simulink model "thermostat"  (R2014b)
settings: Solver=ode1  StartTime=0.0  StopTime=100  FixedStep=0.0001  MaxStep=0.0001  RelTol=1e-3
(part 2 of 2)

== system thermostat/Thermostat44 ==
  Constant : Constant  Value=10
  Constant1 : Constant  Value=37.78
  Discrete-Time Integrator : DiscreteIntegrator  ExternalReset=either  InitialCondition=25  InitialConditionSetting=State (most efficient)  SampleTime=-1
  Discrete-Time Integrator1 : DiscreteIntegrator  ExternalReset=either  InitialCondition=22.78  InitialConditionSetting=State (most efficient)  SampleTime=-1
  MATLAB Function : MATLAB Function  TreatAsAtomicUnit=on
  MATLAB Function1 : MATLAB Function  TreatAsAtomicUnit=on
  Sum : Sum  Inputs=|+-
  Sum1 : Sum  Inputs=|+-
  high : Constant  Value=25
  low : Constant  Value=22.78
  q : Memory
  wires:
  MATLAB Function/1(qNext) -> q/1
  Constant/1 -> Sum/1
  Sum/1 -> Discrete-Time Integrator/1  "x_dot"
  Discrete-Time Integrator1/1 -> MATLAB Function1/2(in1)
  Constant1/1 -> Sum1/1
  Sum1/1 -> Discrete-Time Integrator1/1  "x_dot"
  Discrete-Time Integrator/1 -> MATLAB Function1/1(in0)
  MATLAB Function1/1(out) -> Sum/2, MATLAB Function/1(x), Sum1/2  "x"
  low/1 -> MATLAB Function/3(LOW)
  high/1 -> MATLAB Function/4(HIGH)
  q/1 -> MATLAB Function1/3(ctrl), Discrete-Time Integrator1/2, Discrete-Time Integrator/2, MATLAB Function/2(q)

== system thermostat/Thermostat45 ==
  Constant : Constant  Value=10
  Constant1 : Constant  Value=37.78
  Discrete-Time Integrator : DiscreteIntegrator  ExternalReset=either  InitialCondition=25  InitialConditionSetting=State (most efficient)  SampleTime=-1
  Discrete-Time Integrator1 : DiscreteIntegrator  ExternalReset=either  InitialCondition=22.78  InitialConditionSetting=State (most efficient)  SampleTime=-1
  MATLAB Function : MATLAB Function  TreatAsAtomicUnit=on
  MATLAB Function1 : MATLAB Function  TreatAsAtomicUnit=on
  Sum : Sum  Inputs=|+-
  Sum1 : Sum  Inputs=|+-
  high : Constant  Value=25
  low : Constant  Value=22.78
  q : Memory
  wires:
  MATLAB Function/1(qNext) -> q/1
  Constant/1 -> Sum/1
  Sum/1 -> Discrete-Time Integrator/1  "x_dot"
  Discrete-Time Integrator1/1 -> MATLAB Function1/2(in1)
  Constant1/1 -> Sum1/1
  Sum1/1 -> Discrete-Time Integrator1/1  "x_dot"
  Discrete-Time Integrator/1 -> MATLAB Function1/1(in0)
  MATLAB Function1/1(out) -> Sum/2, MATLAB Function/1(x), Sum1/2  "x"
  low/1 -> MATLAB Function/3(LOW)
  high/1 -> MATLAB Function/4(HIGH)
  q/1 -> MATLAB Function1/3(ctrl), Discrete-Time Integrator1/2, Discrete-Time Integrator/2, MATLAB Function/2(q)

== system thermostat/Thermostat46 ==
  Constant : Constant  Value=10
  Constant1 : Constant  Value=37.78
  Discrete-Time Integrator : DiscreteIntegrator  ExternalReset=either  InitialCondition=25  InitialConditionSetting=State (most efficient)  SampleTime=-1
  Discrete-Time Integrator1 : DiscreteIntegrator  ExternalReset=either  InitialCondition=22.78  InitialConditionSetting=State (most efficient)  SampleTime=-1
  MATLAB Function : MATLAB Function  TreatAsAtomicUnit=on
  MATLAB Function1 : MATLAB Function  TreatAsAtomicUnit=on
  Sum : Sum  Inputs=|+-
  Sum1 : Sum  Inputs=|+-
  high : Constant  Value=25
  low : Constant  Value=22.78
  q : Memory
  wires:
  MATLAB Function/1(qNext) -> q/1
  Constant/1 -> Sum/1
  Sum/1 -> Discrete-Time Integrator/1  "x_dot"
  Discrete-Time Integrator1/1 -> MATLAB Function1/2(in1)
  Constant1/1 -> Sum1/1
  Sum1/1 -> Discrete-Time Integrator1/1  "x_dot"
  Discrete-Time Integrator/1 -> MATLAB Function1/1(in0)
  MATLAB Function1/1(out) -> Sum/2, MATLAB Function/1(x), Sum1/2  "x"
  low/1 -> MATLAB Function/3(LOW)
  high/1 -> MATLAB Function/4(HIGH)
  q/1 -> MATLAB Function1/3(ctrl), Discrete-Time Integrator1/2, Discrete-Time Integrator/2, MATLAB Function/2(q)

== system thermostat/Thermostat47 ==
  Constant : Constant  Value=10
  Constant1 : Constant  Value=37.78
  Discrete-Time Integrator : DiscreteIntegrator  ExternalReset=either  InitialCondition=25  InitialConditionSetting=State (most efficient)  SampleTime=-1
  Discrete-Time Integrator1 : DiscreteIntegrator  ExternalReset=either  InitialCondition=22.78  InitialConditionSetting=State (most efficient)  SampleTime=-1
  MATLAB Function : MATLAB Function  TreatAsAtomicUnit=on
  MATLAB Function1 : MATLAB Function  TreatAsAtomicUnit=on
  Sum : Sum  Inputs=|+-
  Sum1 : Sum  Inputs=|+-
  high : Constant  Value=25
  low : Constant  Value=22.78
  q : Memory
  wires:
  MATLAB Function/1(qNext) -> q/1
  Constant/1 -> Sum/1
  Sum/1 -> Discrete-Time Integrator/1  "x_dot"
  Discrete-Time Integrator1/1 -> MATLAB Function1/2(in1)
  Constant1/1 -> Sum1/1
  Sum1/1 -> Discrete-Time Integrator1/1  "x_dot"
  Discrete-Time Integrator/1 -> MATLAB Function1/1(in0)
  MATLAB Function1/1(out) -> Sum/2, MATLAB Function/1(x), Sum1/2  "x"
  low/1 -> MATLAB Function/3(LOW)
  high/1 -> MATLAB Function/4(HIGH)
  q/1 -> MATLAB Function1/3(ctrl), Discrete-Time Integrator1/2, Discrete-Time Integrator/2, MATLAB Function/2(q)

== system thermostat/Thermostat48 ==
  Constant : Constant  Value=10
  Constant1 : Constant  Value=37.78
  Discrete-Time Integrator : DiscreteIntegrator  ExternalReset=either  InitialCondition=25  InitialConditionSetting=State (most efficient)  SampleTime=-1
  Discrete-Time Integrator1 : DiscreteIntegrator  ExternalReset=either  InitialCondition=22.78  InitialConditionSetting=State (most efficient)  SampleTime=-1
  MATLAB Function : MATLAB Function  TreatAsAtomicUnit=on
  MATLAB Function1 : MATLAB Function  TreatAsAtomicUnit=on
  Sum : Sum  Inputs=|+-
  Sum1 : Sum  Inputs=|+-
  high : Constant  Value=25
  low : Constant  Value=22.78
  q : Memory
  wires:
  MATLAB Function/1(qNext) -> q/1
  Constant/1 -> Sum/1
  Sum/1 -> Discrete-Time Integrator/1  "x_dot"
  Discrete-Time Integrator1/1 -> MATLAB Function1/2(in1)
  Constant1/1 -> Sum1/1
  Sum1/1 -> Discrete-Time Integrator1/1  "x_dot"
  Discrete-Time Integrator/1 -> MATLAB Function1/1(in0)
  MATLAB Function1/1(out) -> Sum/2, MATLAB Function/1(x), Sum1/2  "x"
  low/1 -> MATLAB Function/3(LOW)
  high/1 -> MATLAB Function/4(HIGH)
  q/1 -> MATLAB Function1/3(ctrl), Discrete-Time Integrator1/2, Discrete-Time Integrator/2, MATLAB Function/2(q)

== system thermostat/Thermostat49 ==
  Constant : Constant  Value=10
  Constant1 : Constant  Value=37.78
  Discrete-Time Integrator : DiscreteIntegrator  ExternalReset=either  InitialCondition=25  InitialConditionSetting=State (most efficient)  SampleTime=-1
  Discrete-Time Integrator1 : DiscreteIntegrator  ExternalReset=either  InitialCondition=22.78  InitialConditionSetting=State (most efficient)  SampleTime=-1
  MATLAB Function : MATLAB Function  TreatAsAtomicUnit=on
  MATLAB Function1 : MATLAB Function  TreatAsAtomicUnit=on
  Sum : Sum  Inputs=|+-
  Sum1 : Sum  Inputs=|+-
  high : Constant  Value=25
  low : Constant  Value=22.78
  q : Memory
  wires:
  MATLAB Function/1(qNext) -> q/1
  Constant/1 -> Sum/1
  Sum/1 -> Discrete-Time Integrator/1  "x_dot"
  Discrete-Time Integrator1/1 -> MATLAB Function1/2(in1)
  Constant1/1 -> Sum1/1
  Sum1/1 -> Discrete-Time Integrator1/1  "x_dot"
  Discrete-Time Integrator/1 -> MATLAB Function1/1(in0)
  MATLAB Function1/1(out) -> Sum/2, MATLAB Function/1(x), Sum1/2  "x"
  low/1 -> MATLAB Function/3(LOW)
  high/1 -> MATLAB Function/4(HIGH)
  q/1 -> MATLAB Function1/3(ctrl), Discrete-Time Integrator1/2, Discrete-Time Integrator/2, MATLAB Function/2(q)

== system thermostat/Thermostat5 ==
  Constant : Constant  Value=10
  Constant1 : Constant  Value=37.78
  Discrete-Time Integrator : DiscreteIntegrator  ExternalReset=either  InitialCondition=25  InitialConditionSetting=State (most efficient)  SampleTime=-1
  Discrete-Time Integrator1 : DiscreteIntegrator  ExternalReset=either  InitialCondition=22.78  InitialConditionSetting=State (most efficient)  SampleTime=-1
  MATLAB Function : MATLAB Function  TreatAsAtomicUnit=on
  MATLAB Function1 : MATLAB Function  TreatAsAtomicUnit=on
  Sum : Sum  Inputs=|+-
  Sum1 : Sum  Inputs=|+-
  high : Constant  Value=25
  low : Constant  Value=22.78
  q : Memory
  wires:
  MATLAB Function/1(qNext) -> q/1
  Constant/1 -> Sum/1
  Sum/1 -> Discrete-Time Integrator/1  "x_dot"
  Discrete-Time Integrator1/1 -> MATLAB Function1/2(in1)
  Constant1/1 -> Sum1/1
  Sum1/1 -> Discrete-Time Integrator1/1  "x_dot"
  Discrete-Time Integrator/1 -> MATLAB Function1/1(in0)
  MATLAB Function1/1(out) -> Sum/2, MATLAB Function/1(x), Sum1/2  "x"
  low/1 -> MATLAB Function/3(LOW)
  high/1 -> MATLAB Function/4(HIGH)
  q/1 -> MATLAB Function1/3(ctrl), Discrete-Time Integrator1/2, Discrete-Time Integrator/2, MATLAB Function/2(q)

== system thermostat/Thermostat6 ==
  Constant : Constant  Value=10
  Constant1 : Constant  Value=37.78
  Discrete-Time Integrator : DiscreteIntegrator  ExternalReset=either  InitialCondition=25  InitialConditionSetting=State (most efficient)  SampleTime=-1
  Discrete-Time Integrator1 : DiscreteIntegrator  ExternalReset=either  InitialCondition=22.78  InitialConditionSetting=State (most efficient)  SampleTime=-1
  MATLAB Function : MATLAB Function  TreatAsAtomicUnit=on
  MATLAB Function1 : MATLAB Function  TreatAsAtomicUnit=on
  Sum : Sum  Inputs=|+-
  Sum1 : Sum  Inputs=|+-
  high : Constant  Value=25
  low : Constant  Value=22.78
  q : Memory
  wires:
  MATLAB Function/1(qNext) -> q/1
  Constant/1 -> Sum/1
  Sum/1 -> Discrete-Time Integrator/1  "x_dot"
  Discrete-Time Integrator1/1 -> MATLAB Function1/2(in1)
  Constant1/1 -> Sum1/1
  Sum1/1 -> Discrete-Time Integrator1/1  "x_dot"
  Discrete-Time Integrator/1 -> MATLAB Function1/1(in0)
  MATLAB Function1/1(out) -> Sum/2, MATLAB Function/1(x), Sum1/2  "x"
  low/1 -> MATLAB Function/3(LOW)
  high/1 -> MATLAB Function/4(HIGH)
  q/1 -> MATLAB Function1/3(ctrl), Discrete-Time Integrator1/2, Discrete-Time Integrator/2, MATLAB Function/2(q)

== system thermostat/Thermostat7 ==
  Constant : Constant  Value=10
  Constant1 : Constant  Value=37.78
  Discrete-Time Integrator : DiscreteIntegrator  ExternalReset=either  InitialCondition=25  InitialConditionSetting=State (most efficient)  SampleTime=-1
  Discrete-Time Integrator1 : DiscreteIntegrator  ExternalReset=either  InitialCondition=22.78  InitialConditionSetting=State (most efficient)  SampleTime=-1
  MATLAB Function : MATLAB Function  TreatAsAtomicUnit=on
  MATLAB Function1 : MATLAB Function  TreatAsAtomicUnit=on
  Sum : Sum  Inputs=|+-
  Sum1 : Sum  Inputs=|+-
  high : Constant  Value=25
  low : Constant  Value=22.78
  q : Memory
  wires:
  MATLAB Function/1(qNext) -> q/1
  Constant/1 -> Sum/1
  Sum/1 -> Discrete-Time Integrator/1  "x_dot"
  Discrete-Time Integrator1/1 -> MATLAB Function1/2(in1)
  Constant1/1 -> Sum1/1
  Sum1/1 -> Discrete-Time Integrator1/1  "x_dot"
  Discrete-Time Integrator/1 -> MATLAB Function1/1(in0)
  MATLAB Function1/1(out) -> Sum/2, MATLAB Function/1(x), Sum1/2  "x"
  low/1 -> MATLAB Function/3(LOW)
  high/1 -> MATLAB Function/4(HIGH)
  q/1 -> MATLAB Function1/3(ctrl), Discrete-Time Integrator1/2, Discrete-Time Integrator/2, MATLAB Function/2(q)

== system thermostat/Thermostat8 ==
  Constant : Constant  Value=10
  Constant1 : Constant  Value=37.78
  Discrete-Time Integrator : DiscreteIntegrator  ExternalReset=either  InitialCondition=25  InitialConditionSetting=State (most efficient)  SampleTime=-1
  Discrete-Time Integrator1 : DiscreteIntegrator  ExternalReset=either  InitialCondition=22.78  InitialConditionSetting=State (most efficient)  SampleTime=-1
  MATLAB Function : MATLAB Function  TreatAsAtomicUnit=on
  MATLAB Function1 : MATLAB Function  TreatAsAtomicUnit=on
  Sum : Sum  Inputs=|+-
  Sum1 : Sum  Inputs=|+-
  high : Constant  Value=25
  low : Constant  Value=22.78
  q : Memory
  wires:
  MATLAB Function/1(qNext) -> q/1
  Constant/1 -> Sum/1
  Sum/1 -> Discrete-Time Integrator/1  "x_dot"
  Discrete-Time Integrator1/1 -> MATLAB Function1/2(in1)
  Constant1/1 -> Sum1/1
  Sum1/1 -> Discrete-Time Integrator1/1  "x_dot"
  Discrete-Time Integrator/1 -> MATLAB Function1/1(in0)
  MATLAB Function1/1(out) -> Sum/2, MATLAB Function/1(x), Sum1/2  "x"
  low/1 -> MATLAB Function/3(LOW)
  high/1 -> MATLAB Function/4(HIGH)
  q/1 -> MATLAB Function1/3(ctrl), Discrete-Time Integrator1/2, Discrete-Time Integrator/2, MATLAB Function/2(q)

== system thermostat/Thermostat9 ==
  Constant : Constant  Value=10
  Constant1 : Constant  Value=37.78
  Discrete-Time Integrator : DiscreteIntegrator  ExternalReset=either  InitialCondition=25  InitialConditionSetting=State (most efficient)  SampleTime=-1
  Discrete-Time Integrator1 : DiscreteIntegrator  ExternalReset=either  InitialCondition=22.78  InitialConditionSetting=State (most efficient)  SampleTime=-1
  MATLAB Function : MATLAB Function  TreatAsAtomicUnit=on
  MATLAB Function1 : MATLAB Function  TreatAsAtomicUnit=on
  Sum : Sum  Inputs=|+-
  Sum1 : Sum  Inputs=|+-
  high : Constant  Value=25
  low : Constant  Value=22.78
  q : Memory
  wires:
  MATLAB Function/1(qNext) -> q/1
  Constant/1 -> Sum/1
  Sum/1 -> Discrete-Time Integrator/1  "x_dot"
  Discrete-Time Integrator1/1 -> MATLAB Function1/2(in1)
  Constant1/1 -> Sum1/1
  Sum1/1 -> Discrete-Time Integrator1/1  "x_dot"
  Discrete-Time Integrator/1 -> MATLAB Function1/1(in0)
  MATLAB Function1/1(out) -> Sum/2, MATLAB Function/1(x), Sum1/2  "x"
  low/1 -> MATLAB Function/3(LOW)
  high/1 -> MATLAB Function/4(HIGH)
  q/1 -> MATLAB Function1/3(ctrl), Discrete-Time Integrator1/2, Discrete-Time Integrator/2, MATLAB Function/2(q)

== matlab function thermostat/Thermostat/MATLAB Function1 ==
  data: in0 input; in1 input; ctrl input; out output
function out = select(in0,in1,ctrl)
%#codegen
if(ctrl==0)
    out=in0;
else
    out=in1;
end

== matlab function thermostat/Thermostat/MATLAB Function ==
  data: x input; q input; qNext output; LOW input; HIGH input
function qNext = phi(x,q, LOW, HIGH)
%#codegen
if q==0 && x> LOW
    qNext=0;
elseif q==0 && x <= LOW
    qNext=1;
elseif q==1 && x < HIGH
    qNext=1;
elseif q==1 && x >= HIGH
    qNext=0;
else
    qNext=2; %this should never execute
end

== matlab function thermostat/Thermostat1/MATLAB Function ==
  data: x input; q input; qNext output; LOW input; HIGH input
function qNext = phi(x,q, LOW, HIGH)
%#codegen
if q==0 && x> LOW
    qNext=0;
elseif q==0 && x <= LOW
    qNext=1;
elseif q==1 && x < HIGH
    qNext=1;
elseif q==1 && x >= HIGH
    qNext=0;
else
    qNext=2; %this should never execute
end

== matlab function thermostat/Thermostat1/MATLAB Function1 ==
  data: in0 input; in1 input; ctrl input; out output
function out = select(in0,in1,ctrl)
%#codegen
if(ctrl==0)
    out=in0;
else
    out=in1;
end

== matlab function thermostat/Thermostat2/MATLAB Function ==
  data: x input; q input; qNext output; LOW input; HIGH input
function qNext = phi(x,q, LOW, HIGH)
%#codegen
if q==0 && x> LOW
    qNext=0;
elseif q==0 && x <= LOW
    qNext=1;
elseif q==1 && x < HIGH
    qNext=1;
elseif q==1 && x >= HIGH
    qNext=0;
else
    qNext=2; %this should never execute
end

== matlab function thermostat/Thermostat2/MATLAB Function1 ==
  data: in0 input; in1 input; ctrl input; out output
function out = select(in0,in1,ctrl)
%#codegen
if(ctrl==0)
    out=in0;
else
    out=in1;
end

== matlab function thermostat/Thermostat3/MATLAB Function ==
  data: x input; q input; qNext output; LOW input; HIGH input
function qNext = phi(x,q, LOW, HIGH)
%#codegen
if q==0 && x> LOW
    qNext=0;
elseif q==0 && x <= LOW
    qNext=1;
elseif q==1 && x < HIGH
    qNext=1;
elseif q==1 && x >= HIGH
    qNext=0;
else
    qNext=2; %this should never execute
end

== matlab function thermostat/Thermostat3/MATLAB Function1 ==
  data: in0 input; in1 input; ctrl input; out output
function out = select(in0,in1,ctrl)
%#codegen
if(ctrl==0)
    out=in0;
else
    out=in1;
end

== matlab function thermostat/Thermostat4/MATLAB Function ==
  data: x input; q input; qNext output; LOW input; HIGH input
function qNext = phi(x,q, LOW, HIGH)
%#codegen
if q==0 && x> LOW
    qNext=0;
elseif q==0 && x <= LOW
    qNext=1;
elseif q==1 && x < HIGH
    qNext=1;
elseif q==1 && x >= HIGH
    qNext=0;
else
    qNext=2; %this should never execute
end

== matlab function thermostat/Thermostat4/MATLAB Function1 ==
  data: in0 input; in1 input; ctrl input; out output
function out = select(in0,in1,ctrl)
%#codegen
if(ctrl==0)
    out=in0;
else
    out=in1;
end

== matlab function thermostat/Thermostat5/MATLAB Function ==
  data: x input; q input; qNext output; LOW input; HIGH input
function qNext = phi(x,q, LOW, HIGH)
%#codegen
if q==0 && x> LOW
    qNext=0;
elseif q==0 && x <= LOW
    qNext=1;
elseif q==1 && x < HIGH
    qNext=1;
elseif q==1 && x >= HIGH
    qNext=0;
else
    qNext=2; %this should never execute
end

== matlab function thermostat/Thermostat5/MATLAB Function1 ==
  data: in0 input; in1 input; ctrl input; out output
function out = select(in0,in1,ctrl)
%#codegen
if(ctrl==0)
    out=in0;
else
    out=in1;
end

== matlab function thermostat/Thermostat6/MATLAB Function ==
  data: x input; q input; qNext output; LOW input; HIGH input
function qNext = phi(x,q, LOW, HIGH)
%#codegen
if q==0 && x> LOW
    qNext=0;
elseif q==0 && x <= LOW
    qNext=1;
elseif q==1 && x < HIGH
    qNext=1;
elseif q==1 && x >= HIGH
    qNext=0;
else
    qNext=2; %this should never execute
end

== matlab function thermostat/Thermostat6/MATLAB Function1 ==
  data: in0 input; in1 input; ctrl input; out output
function out = select(in0,in1,ctrl)
%#codegen
if(ctrl==0)
    out=in0;
else
    out=in1;
end

== matlab function thermostat/Thermostat7/MATLAB Function ==
  data: x input; q input; qNext output; LOW input; HIGH input
function qNext = phi(x,q, LOW, HIGH)
%#codegen
if q==0 && x> LOW
    qNext=0;
elseif q==0 && x <= LOW
    qNext=1;
elseif q==1 && x < HIGH
    qNext=1;
elseif q==1 && x >= HIGH
    qNext=0;
else
    qNext=2; %this should never execute
end

== matlab function thermostat/Thermostat7/MATLAB Function1 ==
  data: in0 input; in1 input; ctrl input; out output
function out = select(in0,in1,ctrl)
%#codegen
if(ctrl==0)
    out=in0;
else
    out=in1;
end

== matlab function thermostat/Thermostat8/MATLAB Function ==
  data: x input; q input; qNext output; LOW input; HIGH input
function qNext = phi(x,q, LOW, HIGH)
%#codegen
if q==0 && x> LOW
    qNext=0;
elseif q==0 && x <= LOW
    qNext=1;
elseif q==1 && x < HIGH
    qNext=1;
elseif q==1 && x >= HIGH
    qNext=0;
else
    qNext=2; %this should never execute
end

== matlab function thermostat/Thermostat8/MATLAB Function1 ==
  data: in0 input; in1 input; ctrl input; out output
function out = select(in0,in1,ctrl)
%#codegen
if(ctrl==0)
    out=in0;
else
    out=in1;
end

== matlab function thermostat/Thermostat9/MATLAB Function ==
  data: x input; q input; qNext output; LOW input; HIGH input
function qNext = phi(x,q, LOW, HIGH)
%#codegen
if q==0 && x> LOW
    qNext=0;
elseif q==0 && x <= LOW
    qNext=1;
elseif q==1 && x < HIGH
    qNext=1;
elseif q==1 && x >= HIGH
    qNext=0;
else
    qNext=2; %this should never execute
end

== matlab function thermostat/Thermostat9/MATLAB Function1 ==
  data: in0 input; in1 input; ctrl input; out output
function out = select(in0,in1,ctrl)
%#codegen
if(ctrl==0)
    out=in0;
else
    out=in1;
end

== matlab function thermostat/Thermostat10/MATLAB Function ==
  data: x input; q input; qNext output; LOW input; HIGH input
function qNext = phi(x,q, LOW, HIGH)
%#codegen
if q==0 && x> LOW
    qNext=0;
elseif q==0 && x <= LOW
    qNext=1;
elseif q==1 && x < HIGH
    qNext=1;
elseif q==1 && x >= HIGH
    qNext=0;
else
    qNext=2; %this should never execute
end

== matlab function thermostat/Thermostat10/MATLAB Function1 ==
  data: in0 input; in1 input; ctrl input; out output
function out = select(in0,in1,ctrl)
%#codegen
if(ctrl==0)
    out=in0;
else
    out=in1;
end

== matlab function thermostat/Thermostat11/MATLAB Function ==
  data: x input; q input; qNext output; LOW input; HIGH input
function qNext = phi(x,q, LOW, HIGH)
%#codegen
if q==0 && x> LOW
    qNext=0;
elseif q==0 && x <= LOW
    qNext=1;
elseif q==1 && x < HIGH
    qNext=1;
elseif q==1 && x >= HIGH
    qNext=0;
else
    qNext=2; %this should never execute
end

== matlab function thermostat/Thermostat11/MATLAB Function1 ==
  data: in0 input; in1 input; ctrl input; out output
function out = select(in0,in1,ctrl)
%#codegen
if(ctrl==0)
    out=in0;
else
    out=in1;
end

== matlab function thermostat/Thermostat12/MATLAB Function ==
  data: x input; q input; qNext output; LOW input; HIGH input
function qNext = phi(x,q, LOW, HIGH)
%#codegen
if q==0 && x> LOW
    qNext=0;
elseif q==0 && x <= LOW
    qNext=1;
elseif q==1 && x < HIGH
    qNext=1;
elseif q==1 && x >= HIGH
    qNext=0;
else
    qNext=2; %this should never execute
end

== matlab function thermostat/Thermostat12/MATLAB Function1 ==
  data: in0 input; in1 input; ctrl input; out output
function out = select(in0,in1,ctrl)
%#codegen
if(ctrl==0)
    out=in0;
else
    out=in1;
end

== matlab function thermostat/Thermostat13/MATLAB Function ==
  data: x input; q input; qNext output; LOW input; HIGH input
function qNext = phi(x,q, LOW, HIGH)
%#codegen
if q==0 && x> LOW
    qNext=0;
elseif q==0 && x <= LOW
    qNext=1;
elseif q==1 && x < HIGH
    qNext=1;
elseif q==1 && x >= HIGH
    qNext=0;
else
    qNext=2; %this should never execute
end

== matlab function thermostat/Thermostat13/MATLAB Function1 ==
  data: in0 input; in1 input; ctrl input; out output
function out = select(in0,in1,ctrl)
%#codegen
if(ctrl==0)
    out=in0;
else
    out=in1;
end

== matlab function thermostat/Thermostat14/MATLAB Function ==
  data: x input; q input; qNext output; LOW input; HIGH input
function qNext = phi(x,q, LOW, HIGH)
%#codegen
if q==0 && x> LOW
    qNext=0;
elseif q==0 && x <= LOW
    qNext=1;
elseif q==1 && x < HIGH
    qNext=1;
elseif q==1 && x >= HIGH
    qNext=0;
else
    qNext=2; %this should never execute
end

== matlab function thermostat/Thermostat14/MATLAB Function1 ==
  data: in0 input; in1 input; ctrl input; out output
function out = select(in0,in1,ctrl)
%#codegen
if(ctrl==0)
    out=in0;
else
    out=in1;
end

== matlab function thermostat/Thermostat15/MATLAB Function ==
  data: x input; q input; qNext output; LOW input; HIGH input
function qNext = phi(x,q, LOW, HIGH)
%#codegen
if q==0 && x> LOW
    qNext=0;
elseif q==0 && x <= LOW
    qNext=1;
elseif q==1 && x < HIGH
    qNext=1;
elseif q==1 && x >= HIGH
    qNext=0;
else
    qNext=2; %this should never execute
end

== matlab function thermostat/Thermostat15/MATLAB Function1 ==
  data: in0 input; in1 input; ctrl input; out output
function out = select(in0,in1,ctrl)
%#codegen
if(ctrl==0)
    out=in0;
else
    out=in1;
end

== matlab function thermostat/Thermostat16/MATLAB Function ==
  data: x input; q input; qNext output; LOW input; HIGH input
function qNext = phi(x,q, LOW, HIGH)
%#codegen
if q==0 && x> LOW
    qNext=0;
elseif q==0 && x <= LOW
    qNext=1;
elseif q==1 && x < HIGH
    qNext=1;
elseif q==1 && x >= HIGH
    qNext=0;
else
    qNext=2; %this should never execute
end

== matlab function thermostat/Thermostat16/MATLAB Function1 ==
  data: in0 input; in1 input; ctrl input; out output
function out = select(in0,in1,ctrl)
%#codegen
if(ctrl==0)
    out=in0;
else
    out=in1;
end

== matlab function thermostat/Thermostat17/MATLAB Function ==
  data: x input; q input; qNext output; LOW input; HIGH input
function qNext = phi(x,q, LOW, HIGH)
%#codegen
if q==0 && x> LOW
    qNext=0;
elseif q==0 && x <= LOW
    qNext=1;
elseif q==1 && x < HIGH
    qNext=1;
elseif q==1 && x >= HIGH
    qNext=0;
else
    qNext=2; %this should never execute
end

== matlab function thermostat/Thermostat17/MATLAB Function1 ==
  data: in0 input; in1 input; ctrl input; out output
function out = select(in0,in1,ctrl)
%#codegen
if(ctrl==0)
    out=in0;
else
    out=in1;
end

== matlab function thermostat/Thermostat18/MATLAB Function ==
  data: x input; q input; qNext output; LOW input; HIGH input
function qNext = phi(x,q, LOW, HIGH)
%#codegen
if q==0 && x> LOW
    qNext=0;
elseif q==0 && x <= LOW
    qNext=1;
elseif q==1 && x < HIGH
    qNext=1;
elseif q==1 && x >= HIGH
    qNext=0;
else
    qNext=2; %this should never execute
end

== matlab function thermostat/Thermostat18/MATLAB Function1 ==
  data: in0 input; in1 input; ctrl input; out output
function out = select(in0,in1,ctrl)
%#codegen
if(ctrl==0)
    out=in0;
else
    out=in1;
end

== matlab function thermostat/Thermostat19/MATLAB Function ==
  data: x input; q input; qNext output; LOW input; HIGH input
function qNext = phi(x,q, LOW, HIGH)
%#codegen
if q==0 && x> LOW
    qNext=0;
elseif q==0 && x <= LOW
    qNext=1;
elseif q==1 && x < HIGH
    qNext=1;
elseif q==1 && x >= HIGH
    qNext=0;
else
    qNext=2; %this should never execute
end

== matlab function thermostat/Thermostat19/MATLAB Function1 ==
  data: in0 input; in1 input; ctrl input; out output
function out = select(in0,in1,ctrl)
%#codegen
if(ctrl==0)
    out=in0;
else
    out=in1;
end

== matlab function thermostat/Thermostat20/MATLAB Function ==
  data: x input; q input; qNext output; LOW input; HIGH input
function qNext = phi(x,q, LOW, HIGH)
%#codegen
if q==0 && x> LOW
    qNext=0;
elseif q==0 && x <= LOW
    qNext=1;
elseif q==1 && x < HIGH
    qNext=1;
elseif q==1 && x >= HIGH
    qNext=0;
else
    qNext=2; %this should never execute
end

== matlab function thermostat/Thermostat20/MATLAB Function1 ==
  data: in0 input; in1 input; ctrl input; out output
function out = select(in0,in1,ctrl)
%#codegen
if(ctrl==0)
    out=in0;
else
    out=in1;
end

== matlab function thermostat/Thermostat21/MATLAB Function ==
  data: x input; q input; qNext output; LOW input; HIGH input
function qNext = phi(x,q, LOW, HIGH)
%#codegen
if q==0 && x> LOW
    qNext=0;
elseif q==0 && x <= LOW
    qNext=1;
elseif q==1 && x < HIGH
    qNext=1;
elseif q==1 && x >= HIGH
    qNext=0;
else
    qNext=2; %this should never execute
end

== matlab function thermostat/Thermostat21/MATLAB Function1 ==
  data: in0 input; in1 input; ctrl input; out output
function out = select(in0,in1,ctrl)
%#codegen
if(ctrl==0)
    out=in0;
else
    out=in1;
end

== matlab function thermostat/Thermostat22/MATLAB Function ==
  data: x input; q input; qNext output; LOW input; HIGH input
function qNext = phi(x,q, LOW, HIGH)
%#codegen
if q==0 && x> LOW
    qNext=0;
elseif q==0 && x <= LOW
    qNext=1;
elseif q==1 && x < HIGH
    qNext=1;
elseif q==1 && x >= HIGH
    qNext=0;
else
    qNext=2; %this should never execute
end

== matlab function thermostat/Thermostat22/MATLAB Function1 ==
  data: in0 input; in1 input; ctrl input; out output
function out = select(in0,in1,ctrl)
%#codegen
if(ctrl==0)
    out=in0;
else
    out=in1;
end

== matlab function thermostat/Thermostat23/MATLAB Function ==
  data: x input; q input; qNext output; LOW input; HIGH input
function qNext = phi(x,q, LOW, HIGH)
%#codegen
if q==0 && x> LOW
    qNext=0;
elseif q==0 && x <= LOW
    qNext=1;
elseif q==1 && x < HIGH
    qNext=1;
elseif q==1 && x >= HIGH
    qNext=0;
else
    qNext=2; %this should never execute
end

== matlab function thermostat/Thermostat23/MATLAB Function1 ==
  data: in0 input; in1 input; ctrl input; out output
function out = select(in0,in1,ctrl)
%#codegen
if(ctrl==0)
    out=in0;
else
    out=in1;
end

== matlab function thermostat/Thermostat24/MATLAB Function ==
  data: x input; q input; qNext output; LOW input; HIGH input
function qNext = phi(x,q, LOW, HIGH)
%#codegen
if q==0 && x> LOW
    qNext=0;
elseif q==0 && x <= LOW
    qNext=1;
elseif q==1 && x < HIGH
    qNext=1;
elseif q==1 && x >= HIGH
    qNext=0;
else
    qNext=2; %this should never execute
end

== matlab function thermostat/Thermostat24/MATLAB Function1 ==
  data: in0 input; in1 input; ctrl input; out output
function out = select(in0,in1,ctrl)
%#codegen
if(ctrl==0)
    out=in0;
else
    out=in1;
end

== matlab function thermostat/Thermostat25/MATLAB Function ==
  data: x input; q input; qNext output; LOW input; HIGH input
function qNext = phi(x,q, LOW, HIGH)
%#codegen
if q==0 && x> LOW
    qNext=0;
elseif q==0 && x <= LOW
    qNext=1;
elseif q==1 && x < HIGH
    qNext=1;
elseif q==1 && x >= HIGH
    qNext=0;
else
    qNext=2; %this should never execute
end

== matlab function thermostat/Thermostat25/MATLAB Function1 ==
  data: in0 input; in1 input; ctrl input; out output
function out = select(in0,in1,ctrl)
%#codegen
if(ctrl==0)
    out=in0;
else
    out=in1;
end

== matlab function thermostat/Thermostat26/MATLAB Function ==
  data: x input; q input; qNext output; LOW input; HIGH input
function qNext = phi(x,q, LOW, HIGH)
%#codegen
if q==0 && x> LOW
    qNext=0;
elseif q==0 && x <= LOW
    qNext=1;
elseif q==1 && x < HIGH
    qNext=1;
elseif q==1 && x >= HIGH
    qNext=0;
else
    qNext=2; %this should never execute
end

== matlab function thermostat/Thermostat26/MATLAB Function1 ==
  data: in0 input; in1 input; ctrl input; out output
function out = select(in0,in1,ctrl)
%#codegen
if(ctrl==0)
    out=in0;
else
    out=in1;
end

== matlab function thermostat/Thermostat27/MATLAB Function ==
  data: x input; q input; qNext output; LOW input; HIGH input
function qNext = phi(x,q, LOW, HIGH)
%#codegen
if q==0 && x> LOW
    qNext=0;
elseif q==0 && x <= LOW
    qNext=1;
elseif q==1 && x < HIGH
    qNext=1;
elseif q==1 && x >= HIGH
    qNext=0;
else
    qNext=2; %this should never execute
end

== matlab function thermostat/Thermostat27/MATLAB Function1 ==
  data: in0 input; in1 input; ctrl input; out output
function out = select(in0,in1,ctrl)
%#codegen
if(ctrl==0)
    out=in0;
else
    out=in1;
end

== matlab function thermostat/Thermostat28/MATLAB Function ==
  data: x input; q input; qNext output; LOW input; HIGH input
function qNext = phi(x,q, LOW, HIGH)
%#codegen
if q==0 && x> LOW
    qNext=0;
elseif q==0 && x <= LOW
    qNext=1;
elseif q==1 && x < HIGH
    qNext=1;
elseif q==1 && x >= HIGH
    qNext=0;
else
    qNext=2; %this should never execute
end

== matlab function thermostat/Thermostat28/MATLAB Function1 ==
  data: in0 input; in1 input; ctrl input; out output
function out = select(in0,in1,ctrl)
%#codegen
if(ctrl==0)
    out=in0;
else
    out=in1;
end

== matlab function thermostat/Thermostat29/MATLAB Function ==
  data: x input; q input; qNext output; LOW input; HIGH input
function qNext = phi(x,q, LOW, HIGH)
%#codegen
if q==0 && x> LOW
    qNext=0;
elseif q==0 && x <= LOW
    qNext=1;
elseif q==1 && x < HIGH
    qNext=1;
elseif q==1 && x >= HIGH
    qNext=0;
else
    qNext=2; %this should never execute
end

== matlab function thermostat/Thermostat29/MATLAB Function1 ==
  data: in0 input; in1 input; ctrl input; out output
function out = select(in0,in1,ctrl)
%#codegen
if(ctrl==0)
    out=in0;
else
    out=in1;
end

== matlab function thermostat/Thermostat30/MATLAB Function ==
  data: x input; q input; qNext output; LOW input; HIGH input
function qNext = phi(x,q, LOW, HIGH)
%#codegen
if q==0 && x> LOW
    qNext=0;
elseif q==0 && x <= LOW
    qNext=1;
elseif q==1 && x < HIGH
    qNext=1;
elseif q==1 && x >= HIGH
    qNext=0;
else
    qNext=2; %this should never execute
end

== matlab function thermostat/Thermostat30/MATLAB Function1 ==
  data: in0 input; in1 input; ctrl input; out output
function out = select(in0,in1,ctrl)
%#codegen
if(ctrl==0)
    out=in0;
else
    out=in1;
end

== matlab function thermostat/Thermostat31/MATLAB Function ==
  data: x input; q input; qNext output; LOW input; HIGH input
function qNext = phi(x,q, LOW, HIGH)
%#codegen
if q==0 && x> LOW
    qNext=0;
elseif q==0 && x <= LOW
    qNext=1;
elseif q==1 && x < HIGH
    qNext=1;
elseif q==1 && x >= HIGH
    qNext=0;
else
    qNext=2; %this should never execute
end

== matlab function thermostat/Thermostat31/MATLAB Function1 ==
  data: in0 input; in1 input; ctrl input; out output
function out = select(in0,in1,ctrl)
%#codegen
if(ctrl==0)
    out=in0;
else
    out=in1;
end

== matlab function thermostat/Thermostat32/MATLAB Function ==
  data: x input; q input; qNext output; LOW input; HIGH input
function qNext = phi(x,q, LOW, HIGH)
%#codegen
if q==0 && x> LOW
    qNext=0;
elseif q==0 && x <= LOW
    qNext=1;
elseif q==1 && x < HIGH
    qNext=1;
elseif q==1 && x >= HIGH
    qNext=0;
else
    qNext=2; %this should never execute
end

== matlab function thermostat/Thermostat32/MATLAB Function1 ==
  data: in0 input; in1 input; ctrl input; out output
function out = select(in0,in1,ctrl)
%#codegen
if(ctrl==0)
    out=in0;
else
    out=in1;
end

== matlab function thermostat/Thermostat33/MATLAB Function ==
  data: x input; q input; qNext output; LOW input; HIGH input
function qNext = phi(x,q, LOW, HIGH)
%#codegen
if q==0 && x> LOW
    qNext=0;
elseif q==0 && x <= LOW
    qNext=1;
elseif q==1 && x < HIGH
    qNext=1;
elseif q==1 && x >= HIGH
    qNext=0;
else
    qNext=2; %this should never execute
end

== matlab function thermostat/Thermostat33/MATLAB Function1 ==
  data: in0 input; in1 input; ctrl input; out output
function out = select(in0,in1,ctrl)
%#codegen
if(ctrl==0)
    out=in0;
else
    out=in1;
end

== matlab function thermostat/Thermostat34/MATLAB Function ==
  data: x input; q input; qNext output; LOW input; HIGH input
function qNext = phi(x,q, LOW, HIGH)
%#codegen
if q==0 && x> LOW
    qNext=0;
elseif q==0 && x <= LOW
    qNext=1;
elseif q==1 && x < HIGH
    qNext=1;
elseif q==1 && x >= HIGH
    qNext=0;
else
    qNext=2; %this should never execute
end

== matlab function thermostat/Thermostat34/MATLAB Function1 ==
  data: in0 input; in1 input; ctrl input; out output
function out = select(in0,in1,ctrl)
%#codegen
if(ctrl==0)
    out=in0;
else
    out=in1;
end

== matlab function thermostat/Thermostat35/MATLAB Function ==
  data: x input; q input; qNext output; LOW input; HIGH input
function qNext = phi(x,q, LOW, HIGH)
%#codegen
if q==0 && x> LOW
    qNext=0;
elseif q==0 && x <= LOW
    qNext=1;
elseif q==1 && x < HIGH
    qNext=1;
elseif q==1 && x >= HIGH
    qNext=0;
else
    qNext=2; %this should never execute
end

== matlab function thermostat/Thermostat35/MATLAB Function1 ==
  data: in0 input; in1 input; ctrl input; out output
function out = select(in0,in1,ctrl)
%#codegen
if(ctrl==0)
    out=in0;
else
    out=in1;
end

== matlab function thermostat/Thermostat36/MATLAB Function ==
  data: x input; q input; qNext output; LOW input; HIGH input
function qNext = phi(x,q, LOW, HIGH)
%#codegen
if q==0 && x> LOW
    qNext=0;
elseif q==0 && x <= LOW
    qNext=1;
elseif q==1 && x < HIGH
    qNext=1;
elseif q==1 && x >= HIGH
    qNext=0;
else
    qNext=2; %this should never execute
end

== matlab function thermostat/Thermostat36/MATLAB Function1 ==
  data: in0 input; in1 input; ctrl input; out output
function out = select(in0,in1,ctrl)
%#codegen
if(ctrl==0)
    out=in0;
else
    out=in1;
end

== matlab function thermostat/Thermostat37/MATLAB Function ==
  data: x input; q input; qNext output; LOW input; HIGH input
function qNext = phi(x,q, LOW, HIGH)
%#codegen
if q==0 && x> LOW
    qNext=0;
elseif q==0 && x <= LOW
    qNext=1;
elseif q==1 && x < HIGH
    qNext=1;
elseif q==1 && x >= HIGH
    qNext=0;
else
    qNext=2; %this should never execute
end

== matlab function thermostat/Thermostat37/MATLAB Function1 ==
  data: in0 input; in1 input; ctrl input; out output
function out = select(in0,in1,ctrl)
%#codegen
if(ctrl==0)
    out=in0;
else
    out=in1;
end

== matlab function thermostat/Thermostat38/MATLAB Function ==
  data: x input; q input; qNext output; LOW input; HIGH input
function qNext = phi(x,q, LOW, HIGH)
%#codegen
if q==0 && x> LOW
    qNext=0;
elseif q==0 && x <= LOW
    qNext=1;
elseif q==1 && x < HIGH
    qNext=1;
elseif q==1 && x >= HIGH
    qNext=0;
else
    qNext=2; %this should never execute
end

== matlab function thermostat/Thermostat38/MATLAB Function1 ==
  data: in0 input; in1 input; ctrl input; out output
function out = select(in0,in1,ctrl)
%#codegen
if(ctrl==0)
    out=in0;
else
    out=in1;
end

== matlab function thermostat/Thermostat39/MATLAB Function ==
  data: x input; q input; qNext output; LOW input; HIGH input
function qNext = phi(x,q, LOW, HIGH)
%#codegen
if q==0 && x> LOW
    qNext=0;
elseif q==0 && x <= LOW
    qNext=1;
elseif q==1 && x < HIGH
    qNext=1;
elseif q==1 && x >= HIGH
    qNext=0;
else
    qNext=2; %this should never execute
end

== matlab function thermostat/Thermostat39/MATLAB Function1 ==
  data: in0 input; in1 input; ctrl input; out output
function out = select(in0,in1,ctrl)
%#codegen
if(ctrl==0)
    out=in0;
else
    out=in1;
end

== matlab function thermostat/Thermostat40/MATLAB Function ==
  data: x input; q input; qNext output; LOW input; HIGH input
function qNext = phi(x,q, LOW, HIGH)
%#codegen
if q==0 && x> LOW
    qNext=0;
elseif q==0 && x <= LOW
    qNext=1;
elseif q==1 && x < HIGH
    qNext=1;
elseif q==1 && x >= HIGH
    qNext=0;
else
    qNext=2; %this should never execute
end

== matlab function thermostat/Thermostat40/MATLAB Function1 ==
  data: in0 input; in1 input; ctrl input; out output
function out = select(in0,in1,ctrl)
%#codegen
if(ctrl==0)
    out=in0;
else
    out=in1;
end

== matlab function thermostat/Thermostat41/MATLAB Function ==
  data: x input; q input; qNext output; LOW input; HIGH input
function qNext = phi(x,q, LOW, HIGH)
%#codegen
if q==0 && x> LOW
    qNext=0;
elseif q==0 && x <= LOW
    qNext=1;
elseif q==1 && x < HIGH
    qNext=1;
elseif q==1 && x >= HIGH
    qNext=0;
else
    qNext=2; %this should never execute
end

== matlab function thermostat/Thermostat41/MATLAB Function1 ==
  data: in0 input; in1 input; ctrl input; out output
function out = select(in0,in1,ctrl)
%#codegen
if(ctrl==0)
    out=in0;
else
    out=in1;
end

== matlab function thermostat/Thermostat42/MATLAB Function ==
  data: x input; q input; qNext output; LOW input; HIGH input
function qNext = phi(x,q, LOW, HIGH)
%#codegen
if q==0 && x> LOW
    qNext=0;
elseif q==0 && x <= LOW
    qNext=1;
elseif q==1 && x < HIGH
    qNext=1;
elseif q==1 && x >= HIGH
    qNext=0;
else
    qNext=2; %this should never execute
end

== matlab function thermostat/Thermostat42/MATLAB Function1 ==
  data: in0 input; in1 input; ctrl input; out output
function out = select(in0,in1,ctrl)
%#codegen
if(ctrl==0)
    out=in0;
else
    out=in1;
end

== matlab function thermostat/Thermostat43/MATLAB Function ==
  data: x input; q input; qNext output; LOW input; HIGH input
function qNext = phi(x,q, LOW, HIGH)
%#codegen
if q==0 && x> LOW
    qNext=0;
elseif q==0 && x <= LOW
    qNext=1;
elseif q==1 && x < HIGH
    qNext=1;
elseif q==1 && x >= HIGH
    qNext=0;
else
    qNext=2; %this should never execute
end

== matlab function thermostat/Thermostat43/MATLAB Function1 ==
  data: in0 input; in1 input; ctrl input; out output
function out = select(in0,in1,ctrl)
%#codegen
if(ctrl==0)
    out=in0;
else
    out=in1;
end

== matlab function thermostat/Thermostat44/MATLAB Function ==
  data: x input; q input; qNext output; LOW input; HIGH input
function qNext = phi(x,q, LOW, HIGH)
%#codegen
if q==0 && x> LOW
    qNext=0;
elseif q==0 && x <= LOW
    qNext=1;
elseif q==1 && x < HIGH
    qNext=1;
elseif q==1 && x >= HIGH
    qNext=0;
else
    qNext=2; %this should never execute
end

== matlab function thermostat/Thermostat44/MATLAB Function1 ==
  data: in0 input; in1 input; ctrl input; out output
function out = select(in0,in1,ctrl)
%#codegen
if(ctrl==0)
    out=in0;
else
    out=in1;
end

== matlab function thermostat/Thermostat45/MATLAB Function ==
  data: x input; q input; qNext output; LOW input; HIGH input
function qNext = phi(x,q, LOW, HIGH)
%#codegen
if q==0 && x> LOW
    qNext=0;
elseif q==0 && x <= LOW
    qNext=1;
elseif q==1 && x < HIGH
    qNext=1;
elseif q==1 && x >= HIGH
    qNext=0;
else
    qNext=2; %this should never execute
end

== matlab function thermostat/Thermostat45/MATLAB Function1 ==
  data: in0 input; in1 input; ctrl input; out output
function out = select(in0,in1,ctrl)
%#codegen
if(ctrl==0)
    out=in0;
else
    out=in1;
end

== matlab function thermostat/Thermostat46/MATLAB Function ==
  data: x input; q input; qNext output; LOW input; HIGH input
function qNext = phi(x,q, LOW, HIGH)
%#codegen
if q==0 && x> LOW
    qNext=0;
elseif q==0 && x <= LOW
    qNext=1;
elseif q==1 && x < HIGH
    qNext=1;
elseif q==1 && x >= HIGH
    qNext=0;
else
    qNext=2; %this should never execute
end

== matlab function thermostat/Thermostat46/MATLAB Function1 ==
  data: in0 input; in1 input; ctrl input; out output
function out = select(in0,in1,ctrl)
%#codegen
if(ctrl==0)
    out=in0;
else
    out=in1;
end

== matlab function thermostat/Thermostat47/MATLAB Function ==
  data: x input; q input; qNext output; LOW input; HIGH input
function qNext = phi(x,q, LOW, HIGH)
%#codegen
if q==0 && x> LOW
    qNext=0;
elseif q==0 && x <= LOW
    qNext=1;
elseif q==1 && x < HIGH
    qNext=1;
elseif q==1 && x >= HIGH
    qNext=0;
else
    qNext=2; %this should never execute
end

== matlab function thermostat/Thermostat47/MATLAB Function1 ==
  data: in0 input; in1 input; ctrl input; out output
function out = select(in0,in1,ctrl)
%#codegen
if(ctrl==0)
    out=in0;
else
    out=in1;
end

== matlab function thermostat/Thermostat48/MATLAB Function ==
  data: x input; q input; qNext output; LOW input; HIGH input
function qNext = phi(x,q, LOW, HIGH)
%#codegen
if q==0 && x> LOW
    qNext=0;
elseif q==0 && x <= LOW
    qNext=1;
elseif q==1 && x < HIGH
    qNext=1;
elseif q==1 && x >= HIGH
    qNext=0;
else
    qNext=2; %this should never execute
end

== matlab function thermostat/Thermostat48/MATLAB Function1 ==
  data: in0 input; in1 input; ctrl input; out output
function out = select(in0,in1,ctrl)
%#codegen
if(ctrl==0)
    out=in0;
else
    out=in1;
end

== matlab function thermostat/Thermostat49/MATLAB Function ==
  data: x input; q input; qNext output; LOW input; HIGH input
function qNext = phi(x,q, LOW, HIGH)
%#codegen
if q==0 && x> LOW
    qNext=0;
elseif q==0 && x <= LOW
    qNext=1;
elseif q==1 && x < HIGH
    qNext=1;
elseif q==1 && x >= HIGH
    qNext=0;
else
    qNext=2; %this should never execute
end

== matlab function thermostat/Thermostat49/MATLAB Function1 ==
  data: in0 input; in1 input; ctrl input; out output
function out = select(in0,in1,ctrl)
%#codegen
if(ctrl==0)
    out=in0;
else
    out=in1;
end
